simulink model "DTC"  (R2021b)
settings: Solver=VariableStepAuto  StartTime=0.0  StopTime=10.0  RelTol=1e-3
undefined symbols (not defined in the file): sigbuilder_block
settings Model: Creator=t  LastModifiedBy=t

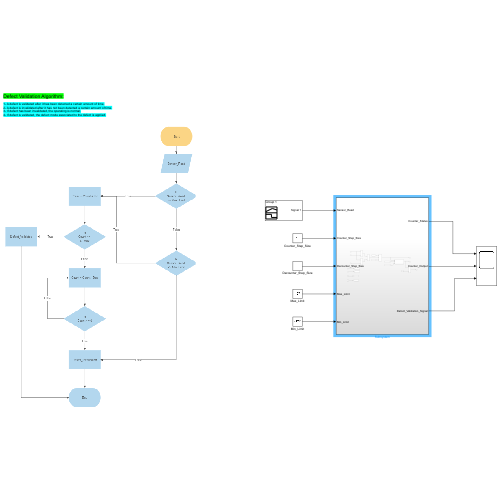
[thumbnail: Simulink's stored preview of the top-level diagram]
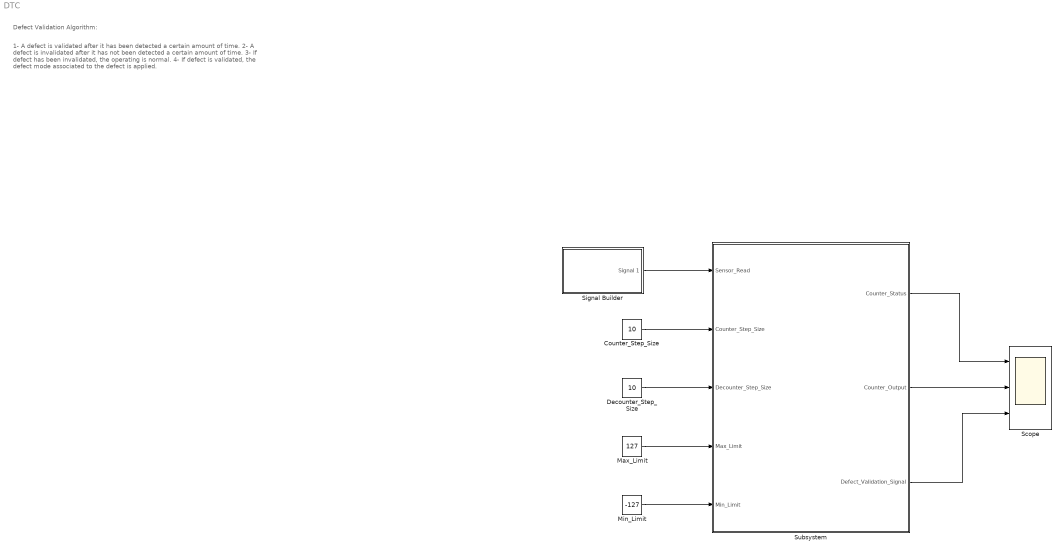
== system DTC ==
  note: 1- A defect is validated after it has been detected a certain amount of time.
      | 2- A defect is invalidated after it has not been detected a certain amount of time.
      | 3- If defect has been invalidated, the operating is normal.
      | 4- If defect is validated, the defect mode associated to the defect is applied.
  note: Defect Validation Algorithm:
  Counter_Step_Size : Constant  Value=10
  Decounter_Step_Size : Constant  Value=10
  Max_Limit : Constant  Value=127
  Min_Limit : Constant  Value=-127
  Scope : Scope  NumInputPorts=3
  Signal Builder : Subsystem  Tag=STV Subsys  LoadFcn=sigbuilder_block('load');  StartFcn=sigbuilder_block('start');  StopFcn=sigbuilder_block('stop');  ClipboardFcn=sigbuilder_block('clipboard');  mask(Sigbuilder block){tuvar=[0:10]}
      mask help: Simulink:masks:SigbuilderBlock_MD
      mask init:
      | if ~strcmp(get_param(bdroot(gcbh),'SimulationStatus'),'stopped') tuvar = sigbuilder_block('maskInit'); end
      settings: CopyFcn=sigbuilder_block('copy');  DeleteFcn=sigbuilder_block('delete');  ModelCloseFcn=sigbuilder_block('modelClose');  PreSaveFcn=sigbuilder_block('preSave');  PauseFcn=sigbuilder_block('pause');  ContinueFcn=sigbuilder_block('continue');  NameChangeFcn=sigbuilder_block('namechange');  OpenFcn=sigbuilder_block('open',[5.4 30 1141.2 522.6 ]);  CloseFcn=sigbuilder_block('close');
      mask Display: plot(0, 0, 100, 100,[2, 2, 32, 32, 2], [68, 8, 8, 68, 68],[32, 2], [38, 38], [32, 19, 2],[53, 60, 44], [32, 17, 17, 2],[16, 16, 31, 31]);txt = getActiveGroup(gcbh);text(2, 100, txt,'verticalAlignment', 'top');
  Subsystem : Subsystem
  wires:
  Signal Builder/1(Signal 1) -> Subsystem/1(Sensor_Read)
  Counter_Step_Size/1 -> Subsystem/2(Counter_Step_Size)
  Decounter_Step_Size/1 -> Subsystem/3(Decounter_Step_Size)
  Subsystem/2(Counter_Output) -> Scope/2
  Subsystem/1(Counter_Status) -> Scope/1
  Subsystem/3(Defect_Validation_Signal) -> Scope/3
  Max_Limit/1 -> Subsystem/4(Max_Limit)
  Min_Limit/1 -> Subsystem/5(Min_Limit)

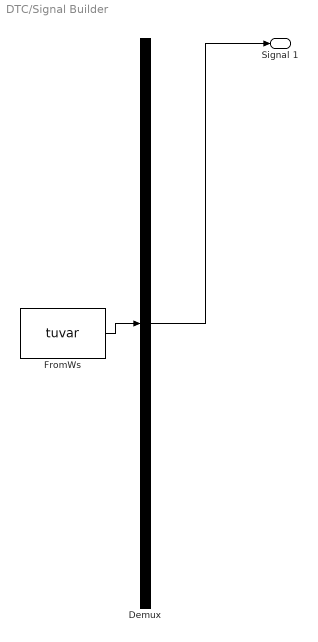
== system DTC/Signal Builder ==
  Demux : Demux  Tag=STV Demux  Outputs=1
      settings: DisplayOption=none
  FromWs : FromWorkspace  Tag=STV FromWs  VariableName=tuvar
      SigBuilderData=|
      | common.afterFinalStr = 'Extrapolate'
      | common.sampleTime = 0
      | dataSet.timeRange = [0 10]
      | dataSet.name = 'Group 1'
      | sbobj.Groups.Name = 'Group 1'
      | sbobj.Groups.Signals.Name = 'Signal 1'
      | sbobj.Groups.Signals.XData = [0 0.35 0.35 3.2 3.2 4 4 7 7 10]
      | sbobj.Groups.Signals.YData = [0 0 100 100 128 128 -100 -100 -129 -129]
  Signal 1 : Outport  Tag=STV Outport
  wires:
  Demux/1 -> Signal 1/1
  FromWs/1 -> Demux/1

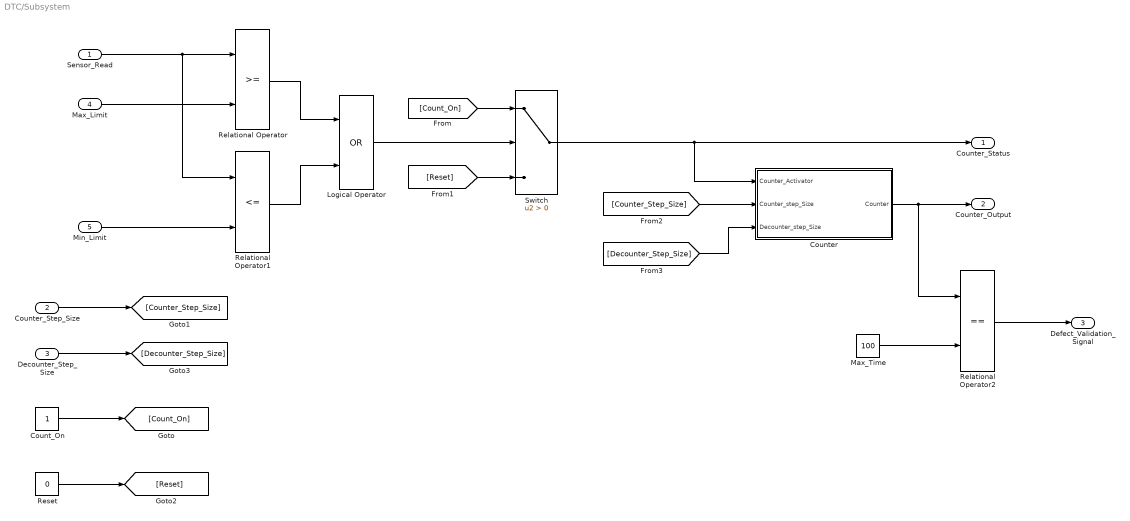
== system DTC/Subsystem ==
  Sensor_Read : Inport
  Counter_Step_Size : Inport  Port=2
  Decounter_Step_Size : Inport  Port=3
  Max_Limit : Inport  Port=4
  Min_Limit : Inport  Port=5
  Count_On : Constant  OutDataTypeStr=Inherit: Inherit via back propagation
  Counter : Subsystem
  Logical Operator : Logic  Operator=OR  AllPortsSameDT=off  OutDataTypeStr=boolean
  Max_Time : Constant  Value=100  OutDataTypeStr=Inherit: Inherit via back propagation
  Relational Operator : RelationalOperator  OutDataTypeStr=boolean  RndMeth=Simplest
  Relational Operator1 : RelationalOperator  Operator=<=  OutDataTypeStr=boolean  RndMeth=Simplest
  Relational Operator2 : RelationalOperator  Operator===  OutDataTypeStr=boolean  RndMeth=Simplest
  Reset : Constant  Value=0  OutDataTypeStr=Inherit: Inherit via back propagation
  Switch : Switch  Criteria=u2 > Threshold
  Counter_Status : Outport
  Counter_Output : Outport  Port=2
  Defect_Validation_Signal : Outport  Port=3
  wires:
  Relational Operator/1 -> Logical Operator/1
  [Count_On] -> Switch/1
  Reset/1 -> [Reset]
  Min_Limit/1 -> Relational Operator1/2
  Relational Operator1/1 -> Logical Operator/2
  Sensor_Read/1 -> Relational Operator/1, Relational Operator1/1
  Logical Operator/1 -> Switch/2
  [Reset] -> Switch/3
  Max_Limit/1 -> Relational Operator/2
  Count_On/1 -> [Count_On]
  Counter_Step_Size/1 -> [Counter_Step_Size]
  Decounter_Step_Size/1 -> [Decounter_Step_Size]
  [Counter_Step_Size] -> Counter/2(Counter_step_Size)
  [Decounter_Step_Size] -> Counter/3(Decounter_step_Size)
  Counter/1(Counter) -> Relational Operator2/1, Counter_Output/1
  Switch/1 -> Counter/1(Counter_Activator), Counter_Status/1
  Max_Time/1 -> Relational Operator2/2
  Relational Operator2/1 -> Defect_Validation_Signal/1

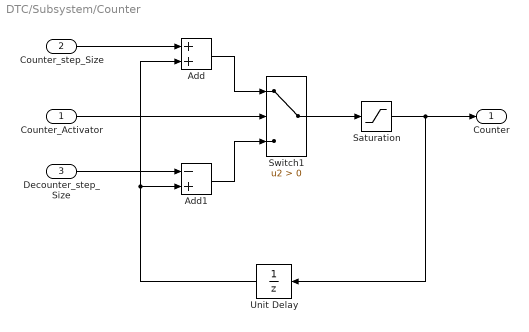
== system DTC/Subsystem/Counter ==
  Counter_Activator : Inport
  Counter_step_Size : Inport  Port=2
  Decounter_step_Size : Inport  Port=3
  Add : Sum
  Add1 : Sum  Inputs=-+
  Saturation : Saturate  UpperLimit=100  LowerLimit=0
  Switch1 : Switch  Criteria=u2 > Threshold
  Unit Delay : UnitDelay  SampleTime=-1  HasFrameUpgradeWarning=on
  Counter : Outport
  wires:
  Counter_step_Size/1 -> Add/1
  Decounter_step_Size/1 -> Add1/1
  Switch1/1 -> Saturation/1
  Unit Delay/1 -> Add/2, Add1/2
  Add1/1 -> Switch1/3
  Add/1 -> Switch1/1
  Counter_Activator/1 -> Switch1/2
  Saturation/1 -> Unit Delay/1, Counter/1
